simulink model "sampleModel1929"  (R2023a)
settings: Solver=VariableStepAuto  StartTime=0.0  StopTime=10.0  RelTol=1e-3
libraries: hdlsllib x4, simulink x2
settings Model: Creator=user1  LastModifiedBy=user1

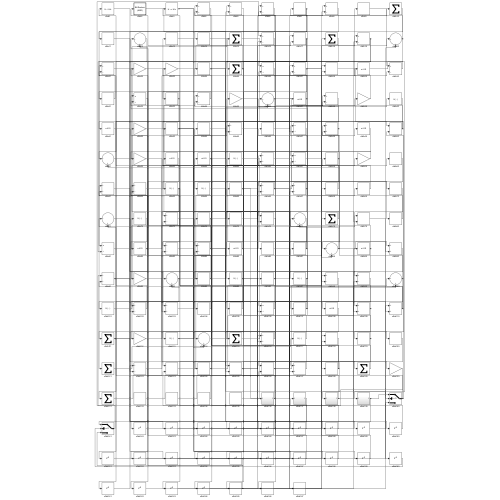
[thumbnail: Simulink's stored preview of the top-level diagram]
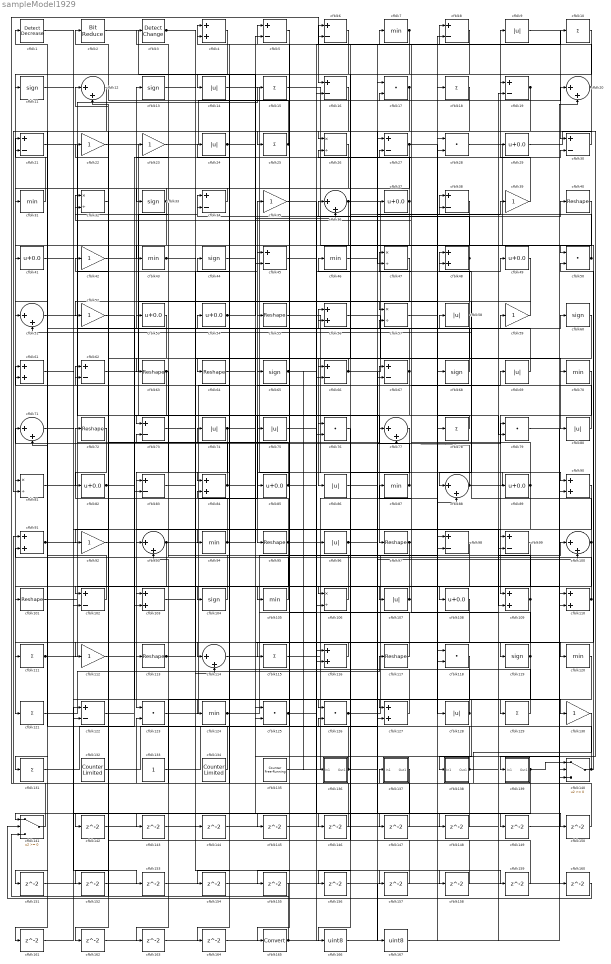
== system sampleModel1929 ==
  cfblk1 : simulink/Logic and Bit Operations/Detect Decrease  vinit=0.0  OutDataTypeStr=boolean
      settings: LibrarySourceBlock=|
      | hdlsllib/Logic and Bit
      | Operations/Detect
      | Decrease
  cfblk{10,15,18,25,78,111,115,121,129,131} (10 alike) : Sum  Inputs=+
  cfblk{12,20,36,51,71,77,88,93,100,114} (10 alike) : Sum  Inputs=|++
  cfblk{40,55,63..64,72,95,97,101,113,117} (10 alike) : Reshape
  cfblk{5..6,8,16,19,21,27,30,34,38,45,62,66..67,73,83,98..99,102,122} (20 alike) : Sum  Inputs=+-
  cfblk{4,48,56,61,84,90..91,103,109..110,116,127} (12 alike) : Sum
  cfblk{11,13,33,44,60,65,68,104,119} (9 alike) : Signum
  cfblk{7,31,43,46,70,87,94,105,120,124} (10 alike) : MinMax
  cfblk{26,32,47,57,81,106} (6 alike) : Product  Inputs=*/  RndMeth=Zero  SaturateOnIntegerOverflow=on
  cfblk{9,14,24,58,69,74..75,80,86,96,107,128} (12 alike) : Abs  SaturateOnIntegerOverflow=off
  cfblk{29,37,41,49,53..54,82,85,89,108} (10 alike) : Bias  Bias=0.0  SaturateOnIntegerOverflow=off
  cfblk{22..23,35,39,42,52,59,92,112,130} (10 alike) : Gain
  cfblk{17,28,50,76,79,118,123,125..126} (9 alike) : DotProduct  OutDataTypeStr=Inherit: Inherit via internal rule
  cfblk132 : hdlsllib/Sources/Counter Limited  uplimit=7  tsamp=-1
  cfblk133 : Constant  SampleTime=-1
  cfblk134 : hdlsllib/Sources/Counter Limited  uplimit=7  tsamp=-1
  cfblk135 : hdlsllib/Sources/Counter Free-Running  NumBits=16  tsamp=-1
  cfblk136 : Subsystem
      settings: LibrarySourceBlock=|
      | hdlsllib/Ports &
      | Subsystems/Subsystem
  cfblk137 : Subsystem
      settings: LibrarySourceBlock=|
      | hdlsllib/Ports &
      | Subsystems/Subsystem
  cfblk138 : Subsystem
      settings: LibrarySourceBlock=|
      | hdlsllib/Ports &
      | Subsystems/Subsystem
  cfblk139 : Subsystem
      settings: LibrarySourceBlock=|
      | hdlsllib/Ports &
      | Subsystems/Subsystem
  cfblk140 : Switch  SaturateOnIntegerOverflow=off  InputSameDT=off
  cfblk141 : Switch  SaturateOnIntegerOverflow=off  InputSameDT=off
  cfblk{142..164} (23 alike) : Delay  SampleTime=1
  cfblk165 : DataTypeConversion  SaturateOnIntegerOverflow=off  RndMeth=Floor
  cfblk166 : DataTypeConversion  OutDataTypeStr=uint8  SaturateOnIntegerOverflow=off  RndMeth=Floor
  cfblk167 : DataTypeConversion  OutDataTypeStr=uint8  SaturateOnIntegerOverflow=off  RndMeth=Floor
  cfblk2 : hdlsllib/Logic and Bit Operations/Bit Reduce  mode=AND
  cfblk3 : simulink/Logic and Bit Operations/Detect Change  vinit=0  OutDataTypeStr=boolean
      settings: LibrarySourceBlock=|
      | hdlsllib/Logic and Bit
      | Operations/Detect
      | Change
  wires:
  cfblk100/1 -> cfblk108/1, cfblk51/2
  cfblk111/1 -> cfblk58/1, cfblk153/1
  cfblk88/1 -> cfblk90/1, cfblk77/2, cfblk48/2
  cfblk4/1 -> cfblk121/1
  cfblk74/1 -> cfblk123/1, cfblk60/1
  cfblk49/1 -> cfblk88/1
  cfblk116/1 -> cfblk112/1
  cfblk15/1 -> cfblk119/1
  cfblk39/1 -> cfblk9/1
  cfblk67/1 -> cfblk95/1, cfblk21/2
  cfblk14/1 -> cfblk90/2
  cfblk58/1 -> cfblk86/1, cfblk48/1
  cfblk135/1 -> cfblk18/1
  cfblk141/1 -> cfblk16/1
  cfblk68/1 -> cfblk13/1
  cfblk48/1 -> cfblk34/1, cfblk152/1
  cfblk66/1 -> cfblk38/1, cfblk130/1, cfblk63/1
  cfblk98/1 -> cfblk141/1
  cfblk78/1 -> cfblk73/1
  cfblk55/1 -> cfblk128/1
  cfblk81/1 -> cfblk15/1
  cfblk123/1 -> cfblk69/1
  cfblk70/1 -> cfblk109/1
  cfblk77/1 -> cfblk126/1
  cfblk62/1 -> cfblk34/2
  cfblk20/1 -> cfblk6/1, cfblk122/2
  cfblk101/1 -> cfblk104/1
  cfblk65/1 -> cfblk136/1(In1), cfblk147/1
  cfblk22/1 -> cfblk97/1
  cfblk29/1 -> cfblk139/1(In1)
  cfblk107/1 -> cfblk106/1, cfblk27/2
  cfblk115/1 -> cfblk89/1
  cfblk124/1 -> cfblk78/1, cfblk24/1
  cfblk8/1 -> cfblk84/1
  cfblk96/1 -> cfblk46/1, cfblk39/1
  cfblk104/1 -> cfblk53/1
  cfblk87/1 -> cfblk23/1, cfblk77/1
  cfblk120/1 -> cfblk138/1(In1)
  cfblk36/1 -> cfblk38/2, cfblk51/1
  cfblk18/1 -> cfblk66/1
  cfblk129/1 -> cfblk5/1
  cfblk94/1 -> cfblk72/1, cfblk56/1
  cfblk93/1 -> cfblk35/1, cfblk101/1
  cfblk28/1 -> cfblk50/1
  cfblk91/1 -> cfblk67/1, cfblk125/2
  cfblk90/1 -> cfblk109/2
  cfblk126/1 -> cfblk68/1, cfblk79/1
  cfblk89/1 -> cfblk103/1, cfblk32/2
  cfblk125/1 -> cfblk127/1, cfblk8/1
  cfblk47/1 -> cfblk114/1
  cfblk60/1 -> cfblk64/1
  cfblk26/1 -> cfblk92/1
  cfblk7/1 -> cfblk26/1, cfblk102/2
  cfblk57/1 -> cfblk28/1
  cfblk128/1 -> cfblk44/1, cfblk61/1
  cfblk56/1 -> cfblk80/1
  cfblk19/1 -> cfblk105/1, cfblk52/1
  cfblk12/1 -> cfblk81/1
  cfblk31/1 -> cfblk21/1
  cfblk6/1 -> cfblk14/1
  cfblk130/1 -> cfblk137/1(In1)
  cfblk33/1 -> cfblk31/1, cfblk151/1
  cfblk117/1 -> cfblk55/1
  cfblk5/1 -> cfblk75/1
  cfblk42/1 -> cfblk88/2
  cfblk133/1 -> cfblk126/2
  cfblk134/1 -> cfblk1/1
  cfblk52/1 -> cfblk129/1
  cfblk25/1 -> cfblk2/1, cfblk155/1
  cfblk63/1 -> cfblk83/1, cfblk103/2
  cfblk97/1 -> cfblk47/1, cfblk162/1
  cfblk17/1 -> cfblk47/2, cfblk45/2, cfblk81/2
  cfblk9/1 -> cfblk30/1
  cfblk23/1 -> cfblk19/1
  cfblk138/1(Out1) -> cfblk65/1, cfblk100/1
  cfblk110/1 -> cfblk36/1, cfblk61/2
  cfblk84/1 -> cfblk71/1, cfblk120/1, cfblk146/1
  cfblk2/1 -> cfblk125/1
  cfblk10/1 -> cfblk11/1
  cfblk72/1 -> cfblk82/1
  cfblk114/1 -> cfblk96/1
  cfblk64/1 -> cfblk76/1
  cfblk21/1 -> cfblk127/2
  cfblk16/1 -> cfblk41/1
  cfblk140/1 -> cfblk50/2, cfblk22/1
  cfblk113/1 -> cfblk59/1, cfblk56/2
  cfblk37/1 -> cfblk85/1, cfblk26/2
  cfblk102/1 -> cfblk71/2
  cfblk27/1 -> cfblk20/1, cfblk115/1, cfblk79/2
  cfblk38/1 -> cfblk131/1
  cfblk121/1 -> cfblk117/1
  cfblk34/1 -> cfblk33/1
  cfblk106/1 -> cfblk32/1
  cfblk3/1 -> cfblk158/1, cfblk159/1
  cfblk108/1 -> cfblk111/1
  cfblk127/1 -> cfblk73/2
  cfblk35/1 -> cfblk99/1
  cfblk136/1(Out1) -> cfblk4/1, cfblk100/2
  cfblk53/1 -> cfblk102/1
  cfblk83/1 -> cfblk114/2
  cfblk50/1 -> cfblk43/1, cfblk4/2
  cfblk82/1 -> cfblk42/1, cfblk29/1
  cfblk118/1 -> cfblk165/1
  cfblk105/1 -> cfblk91/2
  cfblk41/1 -> cfblk93/1
  cfblk45/1 -> cfblk30/2
  cfblk59/1 -> cfblk57/1
  cfblk51/1 -> cfblk5/2
  cfblk122/1 -> cfblk54/1
  cfblk75/1 -> cfblk40/1
  cfblk109/1 -> cfblk113/1, cfblk3/1
  cfblk85/1 -> cfblk62/1, cfblk17/2
  cfblk30/1 -> cfblk25/1
  cfblk1/1 -> cfblk98/2
  cfblk69/1 -> cfblk7/1
  cfblk92/1 -> cfblk107/1
  cfblk103/1 -> cfblk45/1
  cfblk43/1 -> cfblk110/2, cfblk76/2, cfblk157/1
  cfblk54/1 -> cfblk94/1, cfblk36/2
  cfblk46/1 -> cfblk10/1
  cfblk13/1 -> cfblk70/1
  cfblk112/1 -> cfblk74/1
  cfblk132/1 -> cfblk17/1
  cfblk80/1 -> cfblk57/2
  cfblk119/1 -> cfblk87/1, cfblk163/1
  cfblk131/1 -> cfblk83/2
  cfblk139/1(Out1) -> cfblk140/1, cfblk161/1
  cfblk24/1 -> cfblk106/2, cfblk140/2
  cfblk95/1 -> cfblk116/2, cfblk62/2, cfblk49/1, cfblk124/1
  cfblk32/1 -> cfblk142/1
  cfblk142/1 -> cfblk116/1
  cfblk11/1 -> cfblk143/1
  cfblk143/1 -> cfblk19/2
  cfblk73/1 -> cfblk144/1
  cfblk144/1 -> cfblk28/2
  cfblk71/1 -> cfblk145/1
  cfblk145/1 -> cfblk67/2
  cfblk146/1 -> cfblk93/2
  cfblk147/1 -> cfblk91/1
  cfblk44/1 -> cfblk148/1
  cfblk148/1 -> cfblk123/2
  cfblk61/1 -> cfblk149/1
  cfblk149/1 -> cfblk110/1
  cfblk86/1 -> cfblk150/1
  cfblk150/1 -> cfblk84/2
  cfblk151/1 -> cfblk20/2
  cfblk152/1 -> cfblk27/1
  cfblk153/1 -> cfblk8/2
  cfblk40/1 -> cfblk154/1
  cfblk154/1 -> cfblk16/2
  cfblk155/1 -> cfblk141/3
  cfblk76/1 -> cfblk156/1
  cfblk157/1 -> cfblk12/2
  cfblk158/1 -> cfblk98/1
  cfblk159/1 -> cfblk6/2
  cfblk79/1 -> cfblk160/1
  cfblk160/1 -> cfblk141/2
  cfblk161/1 -> cfblk122/1
  cfblk162/1 -> cfblk140/3
  cfblk163/1 -> cfblk99/2
  cfblk137/1(Out1) -> cfblk164/1
  cfblk164/1 -> cfblk66/2
  cfblk165/1 -> cfblk37/1, cfblk12/1
  cfblk99/1 -> cfblk166/1
  cfblk166/1 -> cfblk118/1
  cfblk156/1 -> cfblk167/1
  cfblk167/1 -> cfblk118/2

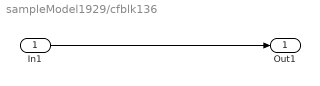
== system sampleModel1929/cfblk136 ==
  In1 : Inport
  Out1 : Outport
  wires:
  In1/1 -> Out1/1

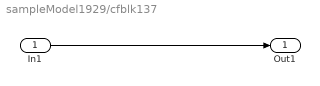
== system sampleModel1929/cfblk137 ==
  In1 : Inport
  Out1 : Outport
  wires:
  In1/1 -> Out1/1

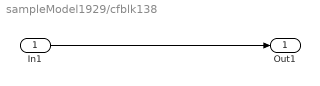
== system sampleModel1929/cfblk138 ==
  In1 : Inport
  Out1 : Outport
  wires:
  In1/1 -> Out1/1

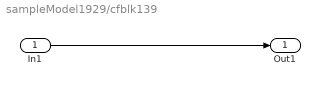
== system sampleModel1929/cfblk139 ==
  In1 : Inport
  Out1 : Outport
  wires:
  In1/1 -> Out1/1
